simulink model "simulation_adaptiveParameters"  (R2016b)
settings: Solver=VariableStepAuto  StartTime=0.0  StopTime=5  RelTol=1e-3
libraries: cstblocks x1
settings Model: Creator=ASUS  LastModifiedBy=ASUS

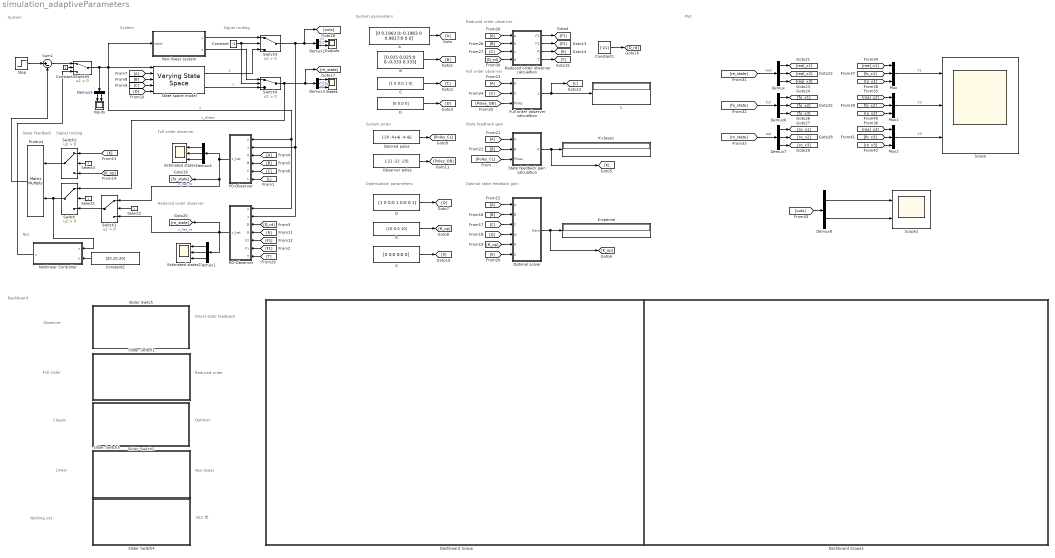
== system simulation_adaptiveParameters ==
  note: NLC
  note: Plot
  note: System
  note: Full order observer
  note: State
      | Feedback
  note: Signal routing
  note: System
  note: State feedback gain
  note: Optimal state feedback gain
  note: Optimization parameters
  note: System poles
  note: Dashboard
  note: Signal routing
  note: Full order observer
  note: System parameters
  note: Reduced order observer
  note: Observer
  note: Direct state
      | feedback
  note: Full order
  note: Reduced order
  note: Classic
  note: Optimal
  note: Linear
  note: Non-linear
  note: Reduced order observer
  note: Nothing yet
  note: NLC 😎
  A : Constant  Value=[0 0.1963 0;-0.1963 0 0.9817;0 0 0]
  B : Constant  Value=[0.025 0.025;0 0;-0.333 0.333]
  C : Constant  Value=[1 0 0;0 1 0]
  Constant : Constant  Value=-1
  Constant1 : Constant  Value=[-21]
  Constant2 : Constant  Value=[20,20,20]
  Constant3 : Constant
  D : Constant  Value=[0 0;0 0]
  Dashboard Scope : Subsystem  DialogController=hmiCreateDDGDialog  IsWebBlock=on  mask(MWDashboardBlock){webBlockId=6c92c294-fc33-4b00-9a21-1f98479c0358, webBlockType=sdiscope, ShowInitialText=on, HMISrcModelName=GeneralModel_2016b}
      mask prompts: webBlockId "WebBlock Id"; webBlockType "WebBlock Type"; HMISrcModelName "Source Model"
      mask help: SimulinkHMI:dialogs:HMIScopeDialogDesc
      mask Help: helpview([docroot '/mapfiles/simulink.map'], 'hmi_scope')
      mask Display:
      | if strcmp(get_param(bdroot(gcb),'BlockDiagramType'), 'library')
      |     image([(matlabroot) '/toolbox/simulink/hmi/icons/DashboardScope.png']);
      | end
  Dashboard Scope1 : Subsystem  DialogController=hmiCreateDDGDialog  IsWebBlock=on  mask(MWDashboardBlock){webBlockId=1342007c-eda9-424f-a5ea-52c521a4ec2e, webBlockType=sdiscope, ShowInitialText=on, HMISrcModelName=GeneralModel_2016b}
      mask prompts: webBlockId "WebBlock Id"; webBlockType "WebBlock Type"; HMISrcModelName "Source Model"
      mask help: SimulinkHMI:dialogs:HMIScopeDialogDesc
      mask Help: helpview([docroot '/mapfiles/simulink.map'], 'hmi_scope')
      mask Display:
      | if strcmp(get_param(bdroot(gcb),'BlockDiagramType'), 'library')
      |     image([(matlabroot) '/toolbox/simulink/hmi/icons/DashboardScope.png']);
      | end
  Demux{,1,3..4,6..7} (6 alike) : Demux  Outputs=3
  Demux2 : Demux  Outputs=2
  Demux5 : Demux  Outputs=2
  Demux8 : Demux  Outputs=2
  Desired poles : Constant  Value=[-20 -4+4j -4-4j]
  Estimated states : Scope  NumInputPorts=3
  Estimated states1 : Scope  NumInputPorts=3
  FO-Observer : Subsystem
  Full order observer calcualtion : MATLAB Function  TreatAsAtomicUnit=on
  Inputs : Scope  NumInputPorts=2
  K-classic : Display
  K-optimal : Display
  L : Display
  Mux : Mux  Inputs=3
  Mux1 : Mux  Inputs=3
  Mux2 : Mux  Inputs=3
  Non-linear system : Subsystem
  Nonlinear Controller : MATLAB Function  TreatAsAtomicUnit=on
  Observer poles : Constant  Value=[-21 -22 -23]
  Optimal solver : MATLAB Function  TreatAsAtomicUnit=on
  Outputs : Scope  NumInputPorts=2
  Product : Product  SCDEnableBlockLinearizationSpecification=on  Multiplication=Matrix(*)
  Q : Constant  Value=[1 0 0;0 1 0;0 0 1]
  R : Constant  Value=[10 0;0 10]
  RO-Observer : Subsystem
  Reduced order observer calcualtion : MATLAB Function  TreatAsAtomicUnit=on
  S : Constant  Value=[0 0;0 0;0 0]
  Scope : Scope  NumInputPorts=3
  Scope1 : Scope  NumInputPorts=2
  Select1 : Constant
  Select2 : Constant
  Select3 : Constant
  Slider Switch : Subsystem  DialogController=hmiCreateDDGDialog  IsWebBlock=on  mask(MWDashboardBlock){webBlockId=44a936f4-a993-4bfe-bf6c-d45eaa0c3901, webBlockType=sliderswitch, ShowInLibBrowser=on, ShowInitialText=on, HMISrcModelName=GeneralModel_2016b}
      mask prompts: webBlockId "WebBlock Id"; webBlockType "WebBlock Type"; HMISrcModelName "Source Model"
      mask help: SimulinkHMI:dialogs:SwitchDialogDesc
      mask Help: helpview([docroot '/mapfiles/simulink.map'], 'hmi_slider_switch')
      mask Display:
      | if strcmp(get_param(bdroot(gcb),'BlockDiagramType'), 'library')
      |     image([(matlabroot) '/toolbox/simulink/hmi/icons/SliderSwitch.png']);
      | end
  Slider Switch1 : Subsystem  DialogController=hmiCreateDDGDialog  IsWebBlock=on  mask(MWDashboardBlock){webBlockId=6f111351-d390-44a2-8560-99747b7fbf3f, webBlockType=sliderswitch, ShowInLibBrowser=on, ShowInitialText=on, HMISrcModelName=GeneralModel_2016b}
      mask prompts: webBlockId "WebBlock Id"; webBlockType "WebBlock Type"; HMISrcModelName "Source Model"
      mask help: SimulinkHMI:dialogs:SwitchDialogDesc
      mask Help: helpview([docroot '/mapfiles/simulink.map'], 'hmi_slider_switch')
      mask Display:
      | if strcmp(get_param(bdroot(gcb),'BlockDiagramType'), 'library')
      |     image([(matlabroot) '/toolbox/simulink/hmi/icons/SliderSwitch.png']);
      | end
  Slider Switch2 : Subsystem  DialogController=hmiCreateDDGDialog  IsWebBlock=on  mask(MWDashboardBlock){webBlockId=37365a62-5cbb-4ea6-bffa-4681a4f0129a, webBlockType=sliderswitch, ShowInLibBrowser=on, ShowInitialText=on, HMISrcModelName=GeneralModel_2016b}
      mask prompts: webBlockId "WebBlock Id"; webBlockType "WebBlock Type"; HMISrcModelName "Source Model"
      mask help: SimulinkHMI:dialogs:SwitchDialogDesc
      mask Help: helpview([docroot '/mapfiles/simulink.map'], 'hmi_slider_switch')
      mask Display:
      | if strcmp(get_param(bdroot(gcb),'BlockDiagramType'), 'library')
      |     image([(matlabroot) '/toolbox/simulink/hmi/icons/SliderSwitch.png']);
      | end
  Slider Switch3 : Subsystem  DialogController=hmiCreateDDGDialog  IsWebBlock=on  mask(MWDashboardBlock){webBlockId=c6c423b7-5d49-4d26-8e58-389c7be099e8, webBlockType=sliderswitch, ShowInLibBrowser=on, ShowInitialText=on, HMISrcModelName=GeneralModel_2016b}
      mask prompts: webBlockId "WebBlock Id"; webBlockType "WebBlock Type"; HMISrcModelName "Source Model"
      mask help: SimulinkHMI:dialogs:SwitchDialogDesc
      mask Help: helpview([docroot '/mapfiles/simulink.map'], 'hmi_slider_switch')
      mask Display:
      | if strcmp(get_param(bdroot(gcb),'BlockDiagramType'), 'library')
      |     image([(matlabroot) '/toolbox/simulink/hmi/icons/SliderSwitch.png']);
      | end
  Slider Switch4 : Subsystem  DialogController=hmiCreateDDGDialog  IsWebBlock=on  mask(MWDashboardBlock){webBlockId=b26f3ce2-438f-4d4a-b8d9-23c156c84292, webBlockType=sliderswitch, ShowInLibBrowser=on, ShowInitialText=on, HMISrcModelName=GeneralModel_2016b}
      mask prompts: webBlockId "WebBlock Id"; webBlockType "WebBlock Type"; HMISrcModelName "Source Model"
      mask help: SimulinkHMI:dialogs:SwitchDialogDesc
      mask Help: helpview([docroot '/mapfiles/simulink.map'], 'hmi_slider_switch')
      mask Display:
      | if strcmp(get_param(bdroot(gcb),'BlockDiagramType'), 'library')
      |     image([(matlabroot) '/toolbox/simulink/hmi/icons/SliderSwitch.png']);
      | end
  State feedback gain calcualtion : MATLAB Function  TreatAsAtomicUnit=on
  State space model : cstblocks/Linear Parameter Varying/Varying State Space  x0=[1;1;1]  xNames=''  OutputX=on  OutputDX=off
  "States " : Scope  NumInputPorts=3
  Step : Step  Time=[1;1]  Before=[1;1]  After=[0;0]  SampleTime=0
  Sum1 : Sum  Inputs=|+-
  Switch{,1..5} (6 alike) : Switch  Criteria=u2 > Threshold
  wires:
  [C] -> State space model/4
  [A] -> State space model/2
  Demux4/3 -> Estimated states/3
  [A] -> FO-Observer/3(A)
  [B] -> FO-Observer/4(B)
  Switch5/1 -> Demux5/1, State space model/1, Non-linear system/1(input), RO-Observer/1(u), FO-Observer/1(u)  "u"
  Demux3/1 -> "States "/1  "x1"
  Demux2/2 -> Outputs/2  "y2"
  Demux3/2 -> "States "/2  "x2"
  [C] -> FO-Observer/5(C)
  FO-Observer/1(x_hat) -> Switch1/1, [fo_state], Demux4/1  "x_hat_fo"
  Demux4/1 -> Estimated states/1
  [D] -> State space model/5
  Demux3/3 -> "States "/3  "x3"
  [B] -> State space model/3
  Mux/1 -> Scope/1  "X1"
  Mux1/1 -> Scope/2  "X2"
  Mux2/1 -> Scope/3  "X3"
  [L] -> FO-Observer/6(L)
  Demux4/2 -> Estimated states/2
  A/1 -> [A]
  B/1 -> [B]
  C/1 -> [C]
  D/1 -> [D]
  Demux2/1 -> Outputs/1  "y1"
  Step/1 -> Sum1/1
  Select1/1 -> Switch/2
  Demux1/2 -> Estimated states1/2
  Demux1/1 -> Estimated states1/1
  [F2] -> RO-Observer/5(F2)
  [R] -> RO-Observer/4(R)
  [D_rd] -> RO-Observer/3(D)
  Demux1/3 -> Estimated states1/3
  RO-Observer/1(x_hat) -> [ro_state], Switch1/3, Demux1/1  "x_hat_ro"
  Select2/1 -> Switch1/2
  Switch1/1 -> Switch/3
  [K] -> Switch2/1
  Select3/1 -> Switch2/2
  [K_op] -> Switch2/3
  State space model/1 -> Switch3/3  "y"
  Switch3/1 -> Demux2/1, [outs], RO-Observer/2(y), FO-Observer/2(y)
  Constant/1 -> Switch3/2, Switch4/2
  Non-linear system/1(y) -> Switch3/1
  Non-linear system/2(x) -> Switch4/1
  Demux5/1 -> Inputs/1
  Demux5/2 -> Inputs/2
  Switch2/1 -> Product/1
  Switch/1 -> Nonlinear Controller/1(x), Product/2
  State space model/2 -> Switch4/3  "x"
  Switch4/1 -> Demux3/1, [re_state], Switch/1  "x_direct"
  Q/1 -> [Q]
  R/1 -> [R_op]
  Optimal solver/1(Gain) -> [K_op], K-optimal/1
  [A] -> Optimal solver/1(A)
  [B] -> Optimal solver/2(B)
  [C] -> Optimal solver/3(C)
  [Q] -> Optimal solver/4(Q)
  [R_op] -> Optimal solver/5(R)
  [S] -> Optimal solver/6(S)
  Desired poles/1 -> [Poles_CL]
  S/1 -> [S]
  Observer poles/1 -> [Poles_OB]
  [B] -> State feedback gain calcualtion/2(B)
  [A] -> State feedback gain calcualtion/1(A)
  [Poles_CL] -> State feedback gain calcualtion/3(Poles)
  State feedback gain calcualtion/1(K) -> K-classic/1, [K]
  [A] -> Full order observer calcualtion/1(A)
  [C] -> Full order observer calcualtion/2(C)
  [Poles_OB] -> Full order observer calcualtion/3(Poles)
  Full order observer calcualtion/1(L) -> [L], L/1
  [A] -> Reduced order observer calcualtion/1(a)
  [C] -> Reduced order observer calcualtion/3(c)
  [B] -> Reduced order observer calcualtion/2(b)
  Reduced order observer calcualtion/1(F1) -> [F1]
  Reduced order observer calcualtion/2(F2) -> [F2]
  Reduced order observer calcualtion/3(R) -> [R]
  Reduced order observer calcualtion/4(T) -> [T]
  [T] -> RO-Observer/7(T)
  [F1] -> RO-Observer/6(F1)
  Constant1/1 -> [D_rd]
  [D_rd] -> Reduced order observer calcualtion/4(d)
  [re_state] -> Demux/1  "real"
  [fo_state] -> Demux6/1  "full"
  [ro_state] -> Demux7/1  "red"
  Demux/1 -> [real_x1]
  Demux/2 -> [real_x2]
  Demux/3 -> [real_x3]
  Demux6/2 -> [fo_x2]
  Demux6/1 -> [fo_x1]
  Demux6/3 -> [fo_x3]
  Demux7/2 -> [ro_x2]
  Demux7/1 -> [ro_x1]
  Demux7/3 -> [ro_x3]
  [real_x1] -> Mux/1
  [real_x2] -> Mux1/1
  [real_x3] -> Mux2/1
  [fo_x1] -> Mux/2
  [ro_x1] -> Mux/3
  [fo_x2] -> Mux1/2
  [ro_x2] -> Mux1/3
  [fo_x3] -> Mux2/2
  [ro_x3] -> Mux2/3
  Demux8/1 -> Scope1/1
  Demux8/2 -> Scope1/2
  [outs] -> Demux8/1
  Constant2/1 -> Nonlinear Controller/2(k)
  Product/1 -> Sum1/2
  Sum1/1 -> Switch5/1
  Nonlinear Controller/1(u) -> Switch5/3
  Constant3/1 -> Switch5/2

== system simulation_adaptiveParameters/Dashboard Scope ==

== system simulation_adaptiveParameters/Dashboard Scope1 ==

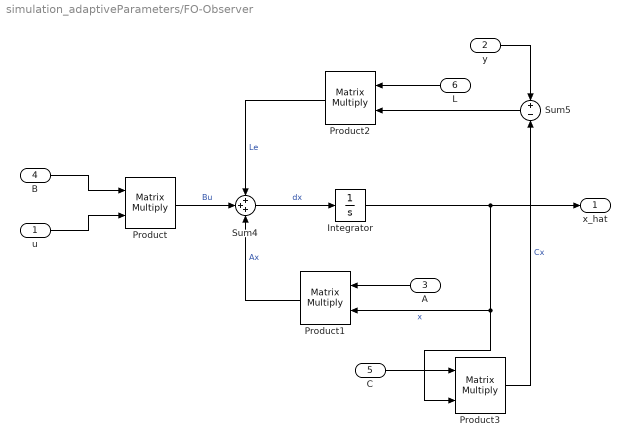
== system simulation_adaptiveParameters/FO-Observer ==
  u : Inport
  y : Inport  Port=2
  A : Inport  Port=3
  B : Inport  Port=4
  C : Inport  Port=5
  L : Inport  Port=6
  Integrator : Integrator  InitialCondition=[0;0;0]
  Product{,1..3} (4 alike) : Product  SCDEnableBlockLinearizationSpecification=on  Multiplication=Matrix(*)
  Sum4 : Sum  Inputs=+++
  Sum5 : Sum  Inputs=+-
  x_hat : Outport
  wires:
  y/1 -> Sum5/1
  Sum5/1 -> Product2/2
  u/1 -> Product/2
  Product3/1 -> Sum5/2  "Cx"
  Sum4/1 -> Integrator/1  "dx"
  Integrator/1 -> x_hat/1, Product1/2, Product3/2  "x"
  C/1 -> Product3/1
  A/1 -> Product1/1
  L/1 -> Product2/1
  B/1 -> Product/1
  Product/1 -> Sum4/2  "Bu"
  Product1/1 -> Sum4/3  "Ax"
  Product2/1 -> Sum4/1  "Le"

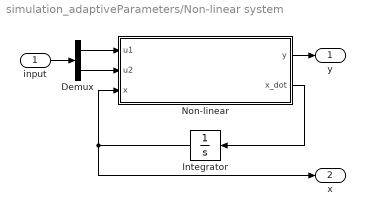
== system simulation_adaptiveParameters/Non-linear system ==
  input : Inport
  Demux : Demux  Outputs=2
  Integrator : Integrator  InitialCondition=[0.05;0.01;0.1]
  Non-linear : MATLAB Function  TreatAsAtomicUnit=on
  y : Outport
  x : Outport  Port=2
  wires:
  Demux/2 -> Non-linear/2(u2)
  Demux/1 -> Non-linear/1(u1)
  input/1 -> Demux/1
  Non-linear/2(x_dot) -> Integrator/1
  Integrator/1 -> Non-linear/3(x), x/1
  Non-linear/1(y) -> y/1

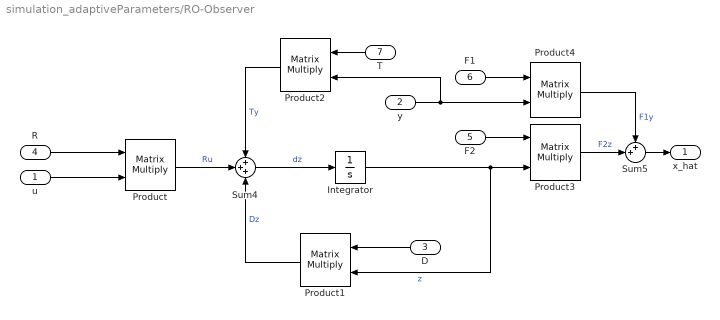
== system simulation_adaptiveParameters/RO-Observer ==
  u : Inport
  y : Inport  Port=2
  D : Inport  Port=3
  R : Inport  Port=4
  F2 : Inport  Port=5
  F1 : Inport  Port=6
  T : Inport  Port=7
  Integrator : Integrator  InitialCondition=[0]
  Product{,1..4} (5 alike) : Product  SCDEnableBlockLinearizationSpecification=on  Multiplication=Matrix(*)
  Sum4 : Sum  Inputs=+++
  Sum5 : Sum  Inputs=++|
  x_hat : Outport
  wires:
  Product2/1 -> Sum4/1  "Ty"
  Product1/1 -> Sum4/3  "Dz"
  Product/1 -> Sum4/2  "Ru"
  R/1 -> Product/1
  D/1 -> Product1/1
  F2/1 -> Product3/1
  Integrator/1 -> Product3/2, Product1/2  "z"
  Sum4/1 -> Integrator/1  "dz"
  u/1 -> Product/2
  Sum5/1 -> x_hat/1
  Product3/1 -> Sum5/2  "F2z"
  y/1 -> Product2/2, Product4/2
  F1/1 -> Product4/1
  Product4/1 -> Sum5/1  "F1y"
  T/1 -> Product2/1

== system simulation_adaptiveParameters/Slider Switch ==

== system simulation_adaptiveParameters/Slider Switch1 ==

== system simulation_adaptiveParameters/Slider Switch2 ==

== system simulation_adaptiveParameters/Slider Switch3 ==

== system simulation_adaptiveParameters/Slider Switch4 ==

== matlab function simulation_adaptiveParameters/Non-linear system/Non-linear ==
  data: u1 input; y output; u2 input; x input; x_dot output
function [y,x_dot] = NLS(u1, u2, x)

Vd = 0.9817;
Wd = 0.1963;

ex = x(1);
ey = x(2);
et = x(3);

ex_dot =  Wd*ey + Vd*(cos(et)-1) - u1*ey + u2;
ey_dot = -Wd*ex + Vd*sin(et)     + u1*ex;
et_dot =  u1;

x_dot = [ex_dot;ey_dot;et_dot];
y = [ex;ey];

== matlab function simulation_adaptiveParameters/Nonlinear Controller ==
  data: x input; u output; k input
function u  = NLC(x,k)
Wr = 0.1963;
Vr = 0.9817;

Vf =  Vr - k(1) * x(1) - Vr * cos(x(3));
Wf = -k(2) * Vr * x(2) - k(3) * sin(x(3));
u = [Vf;Wf];

== matlab function simulation_adaptiveParameters/Optimal solver ==
  data: A input; Gain output; B input; C input; Q input; R input; S input
function Gain = Optim(A,B,C,Q,R,S)

coder.extrinsic('care');

G = zeros(2,3);

% Q = [0.1 0   0
%      0   0.1 0
%      0   0   0.1];
% 
% R = [100 0
%      0  100];
% 
% S = [0 0
%      0 0
%      0 0];
 
E = eye(3);

[P, L, G] = care(A,B,Q,R,S,E);

Gain = G;

== matlab function simulation_adaptiveParameters/State feedback gain calcualtion ==
  data: A input; K output; B input; Poles input
function K = SFB(A,B,Poles)
coder.extrinsic('place');
K = zeros(2,3);
K = place(A,B,Poles)

== matlab function simulation_adaptiveParameters/Full order observer calcualtion ==
  data: A input; L output; C input; Poles input
function L = FOO(A,C,Poles)
coder.extrinsic('place');
L = zeros(3,2);
L = (place(A',C',Poles))'

== matlab function simulation_adaptiveParameters/Reduced order observer calcualtion ==
  data: a input; F1 output; b input; c input; F2 output; R output; T output; d input
function [F1,F2,R,T] = ROO(a,b,c,d)

cq = [0 1 0; 0 0 1];
Q = pinv(c)*cq + [0 0 0;0 0 0;1 0 0];
a_tilda = inv(Q)*a*Q;
a11 = a_tilda(1,1);
a21 = a_tilda(2:3,1);
a12 = a_tilda(1,2:3);
a22 = a_tilda(2:3,2:3);

x = (-21-a11)*pinv(a21);
l2 = x(1,2);
l1 = 1;

T=a12+[l1 l2]*a22 - d*[l1 l2]
lq = [1 l1 l2];
l = lq*inv(Q);
R = l*b
f=inv([c;l]);
F1=f(1:3,1:2)
F2 =f(1:3,3)
